simulink model "check_ndtm"  (R2018b)
settings: configuration reference "Physics" (kept outside this file)
libraries: simulink x1
settings Model: DataDictionary=check_ndtm.sldd  OrderedModelArguments=off  Creator=wischnewski  LastModifiedBy=ga25xiw

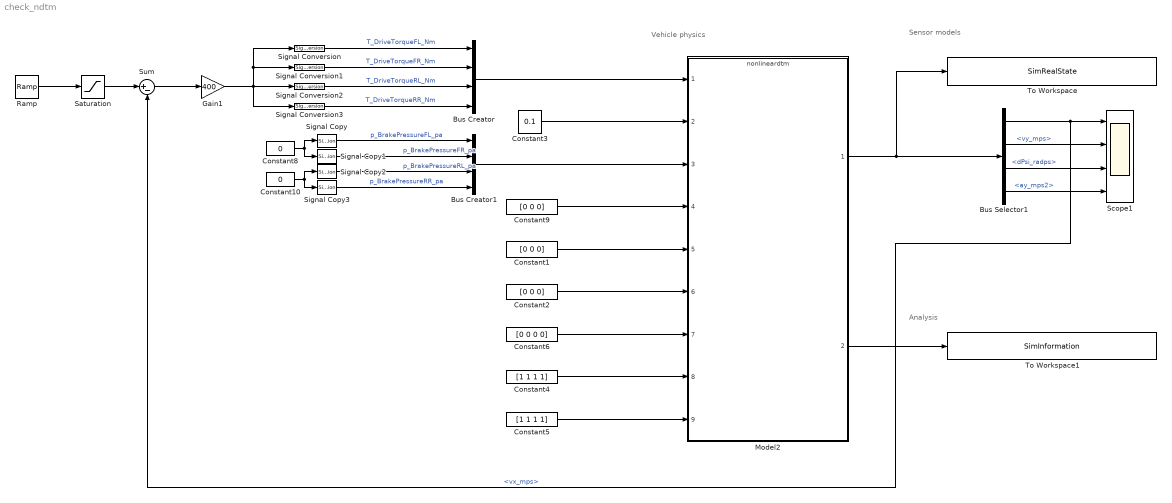
== system check_ndtm ==
  note: Vehicle physics
  note: Analysis
  note: Sensor models
  Bus Creator : BusCreator  Inputs=4  OutDataTypeStr=Bus: DriveTorque_Nm
  Bus Creator1 : BusCreator  Inputs=4  OutDataTypeStr=Bus: BrakePressure_Pa
  Bus Selector1 : BusSelector  OutputSignals=vx_mps,vy_mps,dPsi_radps,ay_mps2
  Constant1 : Constant  Value=[0 0 0]
  Constant10 : Constant  Value=0
  Constant2 : Constant  Value=[0 0 0]
  Constant3 : Constant  Value=0.1
  Constant4 : Constant  Value=[1 1 1 1]
  Constant5 : Constant  Value=[1 1 1 1]
  Constant6 : Constant  Value=[0 0 0 0]
  Constant8 : Constant  Value=0
  Constant9 : Constant  Value=[0 0 0]
  Gain1 : Gain  Gain=400
  Model2 : ModelReference  ModelNameDialog=nonlineardtm  ParameterArgumentNames=x0_initialstates  ParameterArgumentValues=[0 0 0 0 0 -pi/2]  UsingDefaultArgumentValue=0  SimulationMode=Normal  ModelReferenceVersion=1.644
  Ramp : simulink/Sources/Ramp  slope=1  start=0  InitialOutput=0.1
  Saturation : Saturate  UpperLimit=15  LowerLimit=0
  Scope1 : Scope  NumInputPorts=4
  Signal Conversion{,1..3} (4 alike) : SignalConversion  OverrideOpt=off
  Signal Copy{,1..3} (4 alike) : SignalConversion  OverrideOpt=off
  Sum : Sum  Inputs=|+-
  To Workspace : ToWorkspace  VariableName=SimRealState  SaveFormat=Timeseries  SampleTime=-1
  To Workspace1 : ToWorkspace  VariableName=SimInformation  SaveFormat=Timeseries  SampleTime=-1
  wires:
  Model2/1 -> Bus Selector1/1, To Workspace/1
  Constant9/1 -> Model2/4
  Constant1/1 -> Model2/5
  Constant2/1 -> Model2/6
  Model2/2 -> To Workspace1/1
  Constant5/1 -> Model2/9
  Constant6/1 -> Model2/7
  Constant4/1 -> Model2/8
  Ramp/1 -> Saturation/1
  Bus Creator/1 -> Model2/1
  Signal Conversion2/1 -> Bus Creator/3  "T_DriveTorqueRL_Nm"
  Saturation/1 -> Sum/1
  Gain1/1 -> Signal Conversion/1, Signal Conversion1/1, Signal Conversion3/1, Signal Conversion2/1
  Sum/1 -> Gain1/1
  Constant3/1 -> Model2/2
  Signal Conversion3/1 -> Bus Creator/4  "T_DriveTorqueRR_Nm"
  Signal Conversion/1 -> Bus Creator/1  "T_DriveTorqueFL_Nm"
  Signal Conversion1/1 -> Bus Creator/2  "T_DriveTorqueFR_Nm"
  Bus Selector1/1 -> Sum/2, Scope1/1  "<vx_mps>"
  Bus Selector1/4 -> Scope1/4  "<ay_mps2>"
  Bus Selector1/2 -> Scope1/2  "<vy_mps>"
  Bus Selector1/3 -> Scope1/3  "<dPsi_radps>"
  Bus Creator1/1 -> Model2/3
  Signal Copy3/1 -> Bus Creator1/4  "p_BrakePressureRR_pa"
  Constant10/1 -> Signal Copy3/1, Signal Copy2/1
  Constant8/1 -> Signal Copy1/1, Signal Copy/1
  Signal Copy/1 -> Bus Creator1/1  "p_BrakePressureFL_pa"
  Signal Copy2/1 -> Bus Creator1/3  "p_BrakePressureRL_pa"
  Signal Copy1/1 -> Bus Creator1/2  "p_BrakePressureFR_pa"
